simulink model "Dijkstra_Optimization_2"  (R2015b)
settings: Solver=FixedStepDiscrete  SolverMode=SingleTasking  StartTime=0.0  StopTime=10e-5  RelTol=1e-3
libraries: shlslibv1 x995
(part 4 of 6)

== system Dijkstra_Optimization_2/Dijkstra/Subsystem12/Subsystem15/Min_index ==
  dout_sub : Inport
  doutsp_sub : Inport  Port=2
  Comparator1 : shlslibv1/Math Functions/Comparator  syn_comp_opr=a==b  syn_comp_const=on  syn_comp_val=0  syn_en_se=off  synBlockType=primitive  synLatency=0  synBlockId=14
  Comparator2 : shlslibv1/Math Functions/Comparator  syn_comp_opr=a<=b  syn_comp_const=off  syn_comp_val=0  syn_en_se=off  synBlockType=primitive  synLatency=0  synBlockId=14
  Constant4 : shlslibv1/Sources/Constant  syn_cst_val=64  syn_cst_format=Automatic  syn_cst_wl=1  syn_cst_fl=0  syn_cst_dt=unsigned  syn_cst_rnd=on  syn_cst_st=-1  synBlockType=primitive  synLatency=0  synBlockId=15
  Convert1 : shlslibv1/Signal Operations/Convert  syn_preshift_opr=none  syn_preshift_bits=0  syn_preshift_val=0  syn_out_f=Specify  syn_out_wl=64  syn_out_fl=0  syn_out_dt_sync=unsigned  syn_out_sat=off  syn_out_rnd=Floor (Truncate)  syn_inh_port=off  syn_inh_st=off  syn_inh_stf=1  syn_en_pipe=off  syn_pipe_stg=syn_max_pipeline  syn_flow_ctrl=off  syn_sat_op=off  synBlockType=primitive  synLatency=0  synBlockId=4
  Convert2 : shlslibv1/Signal Operations/Convert  syn_preshift_opr=none  syn_preshift_bits=0  syn_preshift_val=0  syn_out_f=Specify  syn_out_wl=4  syn_out_fl=0  syn_out_dt_sync=unsigned  syn_out_sat=off  syn_out_rnd=Floor (Truncate)  syn_inh_port=off  syn_inh_st=off  syn_inh_stf=1  syn_en_pipe=off  syn_pipe_stg=syn_max_pipeline  syn_flow_ctrl=off  syn_sat_op=off  synBlockType=primitive  synLatency=0  synBlockId=4
  Mux : shlslibv1/Signal Operations/Mux  syn_in_nb=2  syn_out_f=Full Precision  syn_out_wl=11  syn_out_fl=52  syn_out_dt=unsigned  syn_en_se=off  synBlockType=primitive  synLatency=0  synBlockId=16
  Switch7 : shlslibv1/Signal Operations/Switch  switchCriteria=u2 != Threshold  switchThresh=0  synBlockType=custom  synLatency=0
  dist10 : shlslibv1/Sources/Sequence  syn_seq_vec=[1 0 0 0 ]  syn_seq_wl=4  syn_seq_fl=0  syn_seq_dt=unsigned  syn_rst_port=off  syn_en_port=off  syn_seq_st=1/(4e6)  synBlockType=custom  synLatency=1
  dist9 : shlslibv1/Sources/Sequence  syn_seq_vec=[0 1 2 3]  syn_seq_wl=4  syn_seq_fl=0  syn_seq_dt=unsigned  syn_rst_port=off  syn_en_port=off  syn_seq_st=1/(4e6)  synBlockType=custom  synLatency=1
  min : shlslibv1/Signal Operations/Mux  syn_in_nb=2  syn_out_f=Full Precision  syn_out_wl=11  syn_out_fl=52  syn_out_dt=unsigned  syn_en_se=off  synBlockType=primitive  synLatency=0  synBlockId=16
  min3 : shlslibv1/Memories/Delay  syn_delay_val=2  synBlockType=primitive  synLatency=2  synBlockId=104
  min4 : shlslibv1/Memories/Delay  syn_delay_val=1  synBlockType=primitive  synLatency=1  synBlockId=104
  min5 : shlslibv1/Memories/Delay  syn_delay_val=1  synBlockType=primitive  synLatency=1  synBlockId=104
  min6 : shlslibv1/Memories/Delay  syn_delay_val=2  synBlockType=primitive  synLatency=2  synBlockId=104
  min_index : shlslibv1/Signal Operations/Mux  syn_in_nb=2  syn_out_f=Full Precision  syn_out_wl=11  syn_out_fl=52  syn_out_dt=unsigned  syn_en_se=off  synBlockType=primitive  synLatency=0  synBlockId=16
  min_sub : Outport
  min_index_sub : Outport  Port=2
  wires:
  min3/1 -> min_index/3
  Comparator1/1 -> Mux/3
  Mux/1 -> Convert2/1
  min/1 -> Convert1/1, min_sub/1
  min_index/1 -> min_index_sub/1, min5/1
  dist9/1 -> min3/1
  dist10/1 -> min6/1
  dout_sub/1 -> Comparator2/1, min/3
  doutsp_sub/1 -> Comparator1/1
  min5/1 -> min_index/2
  Constant4/1 -> Switch7/1
  min6/1 -> Switch7/2
  Switch7/1 -> min/2, Comparator2/2
  min4/1 -> Switch7/3
  Convert2/1 -> min/1, min_index/1
  Convert1/1 -> min4/1
  Comparator2/1 -> Mux/2, Mux/1

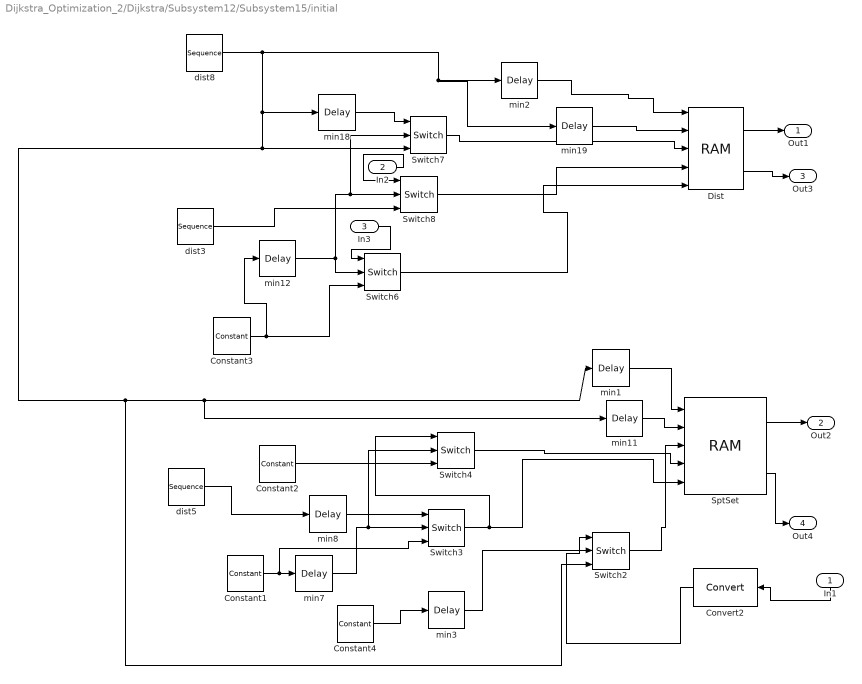
== system Dijkstra_Optimization_2/Dijkstra/Subsystem12/Subsystem15/initial ==
  In1 : Inport
  In2 : Inport  Port=2
  In3 : Inport  Port=3
  Constant1 : shlslibv1/Sources/Constant  syn_cst_val=1  syn_cst_format=Automatic  syn_cst_wl=1  syn_cst_fl=0  syn_cst_dt=unsigned  syn_cst_rnd=on  syn_cst_st=-1  synBlockType=primitive  synLatency=0  synBlockId=15
  Constant2 : shlslibv1/Sources/Constant  syn_cst_val=0  syn_cst_format=Automatic  syn_cst_wl=1  syn_cst_fl=0  syn_cst_dt=unsigned  syn_cst_rnd=on  syn_cst_st=-1  synBlockType=primitive  synLatency=0  synBlockId=15
  Constant3 : shlslibv1/Sources/Constant  syn_cst_val=1  syn_cst_format=Automatic  syn_cst_wl=1  syn_cst_fl=0  syn_cst_dt=unsigned  syn_cst_rnd=on  syn_cst_st=-1  synBlockType=primitive  synLatency=0  synBlockId=15
  Constant4 : shlslibv1/Sources/Constant  syn_cst_val=1  syn_cst_format=Automatic  syn_cst_wl=1  syn_cst_fl=0  syn_cst_dt=unsigned  syn_cst_rnd=on  syn_cst_st=-1  synBlockType=primitive  synLatency=0  synBlockId=15
  Convert2 : shlslibv1/Signal Operations/Convert  syn_preshift_opr=none  syn_preshift_bits=0  syn_preshift_val=0  syn_out_f=Specify  syn_out_wl=4  syn_out_fl=0  syn_out_dt_sync=unsigned  syn_out_sat=off  syn_out_rnd=Floor (Truncate)  syn_inh_port=off  syn_inh_st=off  syn_inh_stf=1  syn_en_pipe=off  syn_pipe_stg=syn_max_pipeline  syn_flow_ctrl=off  syn_sat_op=off  synBlockType=primitive  synLatency=0  synBlockId=4
  "Dist " : shlslibv1/Memories/RAM  syn_ram_depth=4  syn_read_nb=2  syn_write_nb=1  syn_rw_nb=0  syn_corereset=off  syn_localreset=off  syn_initial_val=0  syn_enable_port=off  syn_rrst_port=off  syn_renable_port=off  syn_wac=Write priorization  syn_rac=Cross-port write-first  syn_init_val=0  synBlockType=primitive  synLatency=1  synBlockId=111  syn_spec_init=on
  SptSet : shlslibv1/Memories/RAM  syn_ram_depth=4  syn_read_nb=2  syn_write_nb=1  syn_rw_nb=0  syn_corereset=off  syn_localreset=off  syn_initial_val=0  syn_enable_port=off  syn_rrst_port=off  syn_renable_port=off  syn_wac=Write priorization  syn_rac=Cross-port write-first  syn_init_val=0  synBlockType=primitive  synLatency=1  synBlockId=111  syn_spec_init=on
  Switch{2..4,6..8} (6 alike) : shlslibv1/Signal Operations/Switch  switchCriteria=u2 != Threshold  switchThresh=0  synBlockType=custom  synLatency=0
  dist3 : shlslibv1/Sources/Sequence  syn_seq_vec=[0 64 64 64]  syn_seq_wl=100  syn_seq_fl=0  syn_seq_dt=unsigned  syn_rst_port=off  syn_en_port=off  syn_seq_st=1/(4e6)  synBlockType=custom  synLatency=1
  dist5 : shlslibv1/Sources/Sequence  syn_seq_vec=[0 0 0 1 0 0 0 0 ]  syn_seq_wl=4  syn_seq_fl=0  syn_seq_dt=unsigned  syn_rst_port=off  syn_en_port=off  syn_seq_st=1/(4e6)  synBlockType=custom  synLatency=1
  dist8 : shlslibv1/Sources/Sequence  syn_seq_vec=[0 1 2 3]  syn_seq_wl=4  syn_seq_fl=0  syn_seq_dt=unsigned  syn_rst_port=off  syn_en_port=off  syn_seq_st=1/(4e6)  synBlockType=custom  synLatency=1
  min1 : shlslibv1/Memories/Delay  syn_delay_val=1  synBlockType=primitive  synLatency=1  synBlockId=104
  min{3,7,11..12,19} (5 alike) : shlslibv1/Memories/Delay  syn_delay_val=5  synBlockType=primitive  synLatency=5  synBlockId=104
  min18 : shlslibv1/Memories/Delay  syn_delay_val=6  synBlockType=primitive  synLatency=6  synBlockId=104
  min2 : shlslibv1/Memories/Delay  syn_delay_val=1  synBlockType=primitive  synLatency=1  synBlockId=104
  min8 : shlslibv1/Memories/Delay  syn_delay_val=2  synBlockType=primitive  synLatency=2  synBlockId=104
  Out1 : Outport
  Out2 : Outport  Port=2
  Out3 : Outport  Port=3
  Out4 : Outport  Port=4
  wires:
  In1/1 -> Convert2/1
  In3/1 -> Switch6/1
  In2/1 -> Switch8/1
  min1/1 -> SptSet/1
  min2/1 -> "Dist "/1
  "Dist "/1 -> Out1/1
  SptSet/1 -> Out2/1
  min3/1 -> Switch2/2
  Switch4/1 -> SptSet/4
  Convert2/1 -> Switch2/1
  dist8/1 -> Switch7/3, Switch2/3, min11/1, min1/1, min18/1, min19/1, min2/1
  Constant1/1 -> Switch3/3, min7/1
  Switch3/1 -> Switch4/1, SptSet/5
  Constant2/1 -> Switch4/3
  min7/1 -> Switch4/2, Switch3/2
  dist5/1 -> min8/1
  min8/1 -> Switch3/1
  Switch2/1 -> SptSet/3
  min11/1 -> SptSet/2
  min12/1 -> Switch6/2, Switch8/2, Switch7/2
  Constant3/1 -> Switch6/3, min12/1
  Switch6/1 -> "Dist "/5
  dist3/1 -> Switch8/3
  Switch8/1 -> "Dist "/4
  min18/1 -> Switch7/1
  Switch7/1 -> "Dist "/3
  min19/1 -> "Dist "/2
  Constant4/1 -> min3/1
  SptSet/2 -> Out4/1
  "Dist "/2 -> Out3/1

== system Dijkstra_Optimization_2/Dijkstra/Subsystem12/Subsystem15/min_distance ==
  In1 : Inport
  In2 : Inport  Port=2
  In3 : Inport  Port=3
  In4 : Inport  Port=4
  In5 : Inport  Port=5
  In6 : Inport  Port=6
  In7 : Inport  Port=7
  In8 : Inport  Port=8
  Add1 : shlslibv1/Math Functions/Add  syn_add_opr=++  syn_out_f=Full Precision  syn_out_wl=16  syn_out_fl=8  syn_out_dt=signed  syn_out_sat=off  syn_out_rnd=Floor (Truncate)  synBlockType=primitive  synLatency=0  synBlockId=96  syn_sum_of_rows=off  syn_inh_port=off  syn_inh_st=on  syn_inh_stf=1  syn_en_pipe=off  syn_pipe_stg=syn_max_pipeline  syn_flow_ctrl=off
  Binary Logic1 : shlslibv1/Math Functions/Binary Logic  syn_binlog_exp=a&b&c&d  synBlockType=primitive  synLatency=0  synBlockId=13
  Convert1 : shlslibv1/Signal Operations/Convert  syn_preshift_opr=none  syn_preshift_bits=0  syn_preshift_val=0  syn_out_f=Specify  syn_out_wl=50  syn_out_fl=0  syn_out_dt_sync=unsigned  syn_out_sat=off  syn_out_rnd=Floor (Truncate)  syn_inh_port=off  syn_inh_st=off  syn_inh_stf=1  syn_en_pipe=off  syn_pipe_stg=syn_max_pipeline  syn_flow_ctrl=off  syn_sat_op=off  synBlockType=primitive  synLatency=0  synBlockId=4
  Convert3 : shlslibv1/Signal Operations/Convert  syn_preshift_opr=none  syn_preshift_bits=0  syn_preshift_val=0  syn_out_f=Specify  syn_out_wl=50  syn_out_fl=0  syn_out_dt_sync=unsigned  syn_out_sat=off  syn_out_rnd=Floor (Truncate)  syn_inh_port=off  syn_inh_st=off  syn_inh_stf=1  syn_en_pipe=off  syn_pipe_stg=syn_max_pipeline  syn_flow_ctrl=off  syn_sat_op=off  synBlockType=primitive  synLatency=0  synBlockId=4
  Mux2 : shlslibv1/Signal Operations/Mux  syn_in_nb=4  syn_out_f=Full Precision  syn_out_wl=11  syn_out_fl=52  syn_out_dt=unsigned  syn_en_se=off  synBlockType=primitive  synLatency=0  synBlockId=16
  "dist[u]  INT_MAX " : shlslibv1/Math Functions/Comparator  syn_comp_opr=a!=b  syn_comp_const=on  syn_comp_val=64  syn_en_se=off  synBlockType=primitive  synLatency=0  synBlockId=14
  dist[u][u][v]  dist[v] : shlslibv1/Math Functions/Comparator  syn_comp_opr=a<b  syn_comp_const=off  syn_comp_val=64  syn_en_se=off  synBlockType=primitive  synLatency=0  synBlockId=14
  graph[u][v] : shlslibv1/Math Functions/Comparator  syn_comp_opr=a!=b  syn_comp_const=on  syn_comp_val=0  syn_en_se=off  synBlockType=primitive  synLatency=0  synBlockId=14
  "v]\t" : shlslibv1/Math Functions/Comparator  syn_comp_opr=a==b  syn_comp_const=on  syn_comp_val=0  syn_en_se=off  synBlockType=primitive  synLatency=0  synBlockId=14
  Out1 : Outport
  Out2 : Outport  Port=2
  wires:
  In5/1 -> Mux2/2
  In6/1 -> Mux2/3
  dist[u][u][v]  dist[v]/1 -> Binary Logic1/1
  "dist[u]  INT_MAX "/1 -> Binary Logic1/2
  graph[u][v]/1 -> Binary Logic1/3
  Add1/1 -> Convert3/1, dist[u][u][v]  dist[v]/1
  Binary Logic1/1 -> Convert1/1
  "v]\t"/1 -> Binary Logic1/4
  Mux2/1 -> Add1/2, graph[u][v]/1
  In4/1 -> "v]\t"/1
  Convert3/1 -> Out1/1
  Convert1/1 -> Out2/1
  In1/1 -> dist[u][u][v]  dist[v]/2
  In2/1 -> "dist[u]  INT_MAX "/1, Add1/1
  In3/1 -> Mux2/1
  In8/1 -> Mux2/5
  In7/1 -> Mux2/4

== system Dijkstra_Optimization_2/Dijkstra/Subsystem13/Subsystem16/Delay ==
  In1 : Inport
  In2 : Inport  Port=2
  Switch10 : shlslibv1/Signal Operations/Switch  switchCriteria=u2 != Threshold  switchThresh=0  synBlockType=custom  synLatency=0
  Switch5 : shlslibv1/Signal Operations/Switch  switchCriteria=u2 != Threshold  switchThresh=0  synBlockType=custom  synLatency=0
  dist6 : shlslibv1/Sources/Sequence  syn_seq_vec=[0 0 0 1 0 0 0 0 ]  syn_seq_wl=4  syn_seq_fl=0  syn_seq_dt=unsigned  syn_rst_port=off  syn_en_port=off  syn_seq_st=1/(4e6)  synBlockType=custom  synLatency=1
  min10 : shlslibv1/Memories/Delay  syn_delay_val=2  synBlockType=primitive  synLatency=2  synBlockId=104
  min4 : shlslibv1/Memories/Delay  syn_delay_val=1  synBlockType=primitive  synLatency=1  synBlockId=104
  min9 : shlslibv1/Memories/Delay  syn_delay_val=1  synBlockType=primitive  synLatency=1  synBlockId=104
  Out1 : Outport
  Out2 : Outport  Port=2
  wires:
  In2/1 -> Switch5/1
  dist6/1 -> min10/1
  min10/1 -> Switch5/2, Switch10/2
  In1/1 -> Switch10/1
  Switch10/1 -> Out1/1, min9/1
  Switch5/1 -> min4/1
  min9/1 -> Switch10/3
  min4/1 -> Switch5/3, Out2/1

== system Dijkstra_Optimization_2/Dijkstra/Subsystem13/Subsystem16/Input ==
  In1 : Inport
  In2 : Inport  Port=2
  In3 : Inport  Port=3
  In4 : Inport  Port=4
  Constant5 : shlslibv1/Sources/Constant  syn_cst_val=1  syn_cst_format=Automatic  syn_cst_wl=1  syn_cst_fl=0  syn_cst_dt=unsigned  syn_cst_rnd=on  syn_cst_st=-1  synBlockType=primitive  synLatency=0  synBlockId=15
  Constant6 : shlslibv1/Sources/Constant  syn_cst_val=0  syn_cst_format=Automatic  syn_cst_wl=1  syn_cst_fl=0  syn_cst_dt=unsigned  syn_cst_rnd=on  syn_cst_st=-1  synBlockType=primitive  synLatency=0  synBlockId=15
  Graph{0..3} (4 alike) : shlslibv1/Memories/RAM  syn_ram_depth=4  syn_read_nb=1  syn_write_nb=1  syn_rw_nb=0  syn_corereset=off  syn_localreset=off  syn_initial_val=0  syn_enable_port=off  syn_rrst_port=off  syn_renable_port=off  syn_wac=Write priorization  syn_rac=Cross-port write-first  syn_init_val=0  synBlockType=primitive  synLatency=1  synBlockId=111  syn_spec_init=on
  Switch1 : shlslibv1/Signal Operations/Switch  switchCriteria=u2 != Threshold  switchThresh=0  synBlockType=custom  synLatency=0
  dist9 : shlslibv1/Sources/Sequence  syn_seq_vec=[0 1 2 3 ]  syn_seq_wl=4  syn_seq_fl=0  syn_seq_dt=unsigned  syn_rst_port=off  syn_en_port=off  syn_seq_st=1/(4e6)  synBlockType=custom  synLatency=1
  min14 : shlslibv1/Memories/Delay  syn_delay_val=5  synBlockType=primitive  synLatency=5  synBlockId=104
  min15 : shlslibv1/Memories/Delay  syn_delay_val=5  synBlockType=primitive  synLatency=5  synBlockId=104
  Out1 : Outport
  Out2 : Outport  Port=2
  Out3 : Outport  Port=3
  Out4 : Outport  Port=4
  wires:
  Constant5/1 -> min14/1, Switch1/3
  min14/1 -> Switch1/2
  Switch1/1 -> Graph3/4, Graph2/4, Graph1/4, Graph0/4
  Constant6/1 -> Switch1/1
  In1/1 -> Graph0/3
  In2/1 -> Graph1/3
  In3/1 -> Graph2/3
  In4/1 -> Graph3/3
  dist9/1 -> min15/1, Graph3/2, Graph2/2, Graph1/2, Graph0/2
  min15/1 -> Graph2/1, Graph3/1, Graph1/1, Graph0/1
  Graph0/1 -> Out1/1
  Graph3/1 -> Out4/1
  Graph2/1 -> Out3/1
  Graph1/1 -> Out2/1

== system Dijkstra_Optimization_2/Dijkstra/Subsystem13/Subsystem16/Min_index ==
  dout_sub : Inport
  doutsp_sub : Inport  Port=2
  Comparator1 : shlslibv1/Math Functions/Comparator  syn_comp_opr=a==b  syn_comp_const=on  syn_comp_val=0  syn_en_se=off  synBlockType=primitive  synLatency=0  synBlockId=14
  Comparator2 : shlslibv1/Math Functions/Comparator  syn_comp_opr=a<=b  syn_comp_const=off  syn_comp_val=0  syn_en_se=off  synBlockType=primitive  synLatency=0  synBlockId=14
  Constant4 : shlslibv1/Sources/Constant  syn_cst_val=64  syn_cst_format=Automatic  syn_cst_wl=1  syn_cst_fl=0  syn_cst_dt=unsigned  syn_cst_rnd=on  syn_cst_st=-1  synBlockType=primitive  synLatency=0  synBlockId=15
  Convert1 : shlslibv1/Signal Operations/Convert  syn_preshift_opr=none  syn_preshift_bits=0  syn_preshift_val=0  syn_out_f=Specify  syn_out_wl=64  syn_out_fl=0  syn_out_dt_sync=unsigned  syn_out_sat=off  syn_out_rnd=Floor (Truncate)  syn_inh_port=off  syn_inh_st=off  syn_inh_stf=1  syn_en_pipe=off  syn_pipe_stg=syn_max_pipeline  syn_flow_ctrl=off  syn_sat_op=off  synBlockType=primitive  synLatency=0  synBlockId=4
  Convert2 : shlslibv1/Signal Operations/Convert  syn_preshift_opr=none  syn_preshift_bits=0  syn_preshift_val=0  syn_out_f=Specify  syn_out_wl=4  syn_out_fl=0  syn_out_dt_sync=unsigned  syn_out_sat=off  syn_out_rnd=Floor (Truncate)  syn_inh_port=off  syn_inh_st=off  syn_inh_stf=1  syn_en_pipe=off  syn_pipe_stg=syn_max_pipeline  syn_flow_ctrl=off  syn_sat_op=off  synBlockType=primitive  synLatency=0  synBlockId=4
  Mux : shlslibv1/Signal Operations/Mux  syn_in_nb=2  syn_out_f=Full Precision  syn_out_wl=11  syn_out_fl=52  syn_out_dt=unsigned  syn_en_se=off  synBlockType=primitive  synLatency=0  synBlockId=16
  Switch7 : shlslibv1/Signal Operations/Switch  switchCriteria=u2 != Threshold  switchThresh=0  synBlockType=custom  synLatency=0
  dist10 : shlslibv1/Sources/Sequence  syn_seq_vec=[1 0 0 0 ]  syn_seq_wl=4  syn_seq_fl=0  syn_seq_dt=unsigned  syn_rst_port=off  syn_en_port=off  syn_seq_st=1/(4e6)  synBlockType=custom  synLatency=1
  dist9 : shlslibv1/Sources/Sequence  syn_seq_vec=[0 1 2 3]  syn_seq_wl=4  syn_seq_fl=0  syn_seq_dt=unsigned  syn_rst_port=off  syn_en_port=off  syn_seq_st=1/(4e6)  synBlockType=custom  synLatency=1
  min : shlslibv1/Signal Operations/Mux  syn_in_nb=2  syn_out_f=Full Precision  syn_out_wl=11  syn_out_fl=52  syn_out_dt=unsigned  syn_en_se=off  synBlockType=primitive  synLatency=0  synBlockId=16
  min3 : shlslibv1/Memories/Delay  syn_delay_val=2  synBlockType=primitive  synLatency=2  synBlockId=104
  min4 : shlslibv1/Memories/Delay  syn_delay_val=1  synBlockType=primitive  synLatency=1  synBlockId=104
  min5 : shlslibv1/Memories/Delay  syn_delay_val=1  synBlockType=primitive  synLatency=1  synBlockId=104
  min6 : shlslibv1/Memories/Delay  syn_delay_val=2  synBlockType=primitive  synLatency=2  synBlockId=104
  min_index : shlslibv1/Signal Operations/Mux  syn_in_nb=2  syn_out_f=Full Precision  syn_out_wl=11  syn_out_fl=52  syn_out_dt=unsigned  syn_en_se=off  synBlockType=primitive  synLatency=0  synBlockId=16
  min_sub : Outport
  min_index_sub : Outport  Port=2
  wires:
  min3/1 -> min_index/3
  Comparator1/1 -> Mux/3
  Mux/1 -> Convert2/1
  min/1 -> Convert1/1, min_sub/1
  min_index/1 -> min_index_sub/1, min5/1
  dist9/1 -> min3/1
  dist10/1 -> min6/1
  dout_sub/1 -> Comparator2/1, min/3
  doutsp_sub/1 -> Comparator1/1
  min5/1 -> min_index/2
  Constant4/1 -> Switch7/1
  min6/1 -> Switch7/2
  Switch7/1 -> min/2, Comparator2/2
  min4/1 -> Switch7/3
  Convert2/1 -> min/1, min_index/1
  Convert1/1 -> min4/1
  Comparator2/1 -> Mux/2, Mux/1

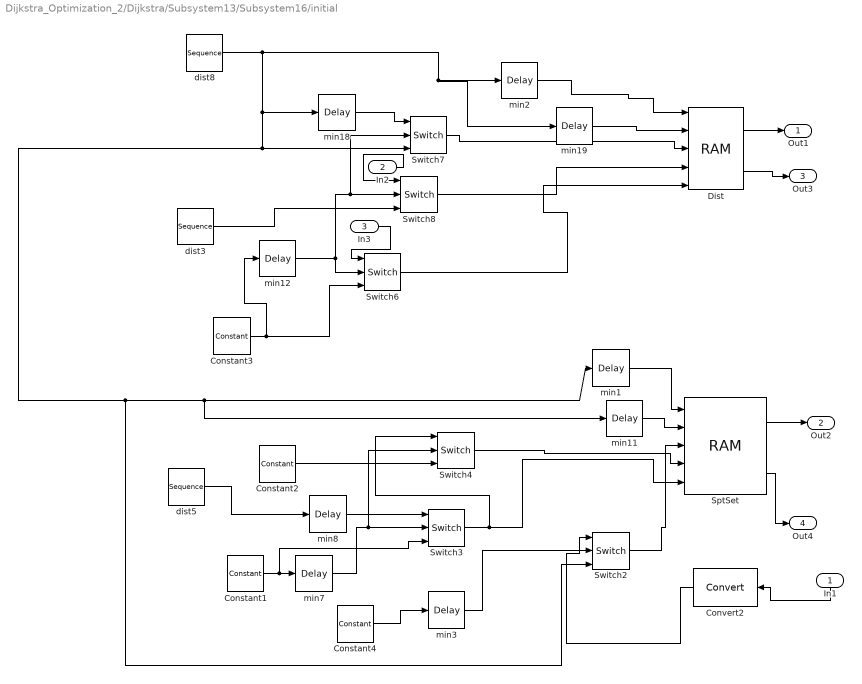
== system Dijkstra_Optimization_2/Dijkstra/Subsystem13/Subsystem16/initial ==
  In1 : Inport
  In2 : Inport  Port=2
  In3 : Inport  Port=3
  Constant1 : shlslibv1/Sources/Constant  syn_cst_val=1  syn_cst_format=Automatic  syn_cst_wl=1  syn_cst_fl=0  syn_cst_dt=unsigned  syn_cst_rnd=on  syn_cst_st=-1  synBlockType=primitive  synLatency=0  synBlockId=15
  Constant2 : shlslibv1/Sources/Constant  syn_cst_val=0  syn_cst_format=Automatic  syn_cst_wl=1  syn_cst_fl=0  syn_cst_dt=unsigned  syn_cst_rnd=on  syn_cst_st=-1  synBlockType=primitive  synLatency=0  synBlockId=15
  Constant3 : shlslibv1/Sources/Constant  syn_cst_val=1  syn_cst_format=Automatic  syn_cst_wl=1  syn_cst_fl=0  syn_cst_dt=unsigned  syn_cst_rnd=on  syn_cst_st=-1  synBlockType=primitive  synLatency=0  synBlockId=15
  Constant4 : shlslibv1/Sources/Constant  syn_cst_val=1  syn_cst_format=Automatic  syn_cst_wl=1  syn_cst_fl=0  syn_cst_dt=unsigned  syn_cst_rnd=on  syn_cst_st=-1  synBlockType=primitive  synLatency=0  synBlockId=15
  Convert2 : shlslibv1/Signal Operations/Convert  syn_preshift_opr=none  syn_preshift_bits=0  syn_preshift_val=0  syn_out_f=Specify  syn_out_wl=4  syn_out_fl=0  syn_out_dt_sync=unsigned  syn_out_sat=off  syn_out_rnd=Floor (Truncate)  syn_inh_port=off  syn_inh_st=off  syn_inh_stf=1  syn_en_pipe=off  syn_pipe_stg=syn_max_pipeline  syn_flow_ctrl=off  syn_sat_op=off  synBlockType=primitive  synLatency=0  synBlockId=4
  "Dist " : shlslibv1/Memories/RAM  syn_ram_depth=4  syn_read_nb=2  syn_write_nb=1  syn_rw_nb=0  syn_corereset=off  syn_localreset=off  syn_initial_val=0  syn_enable_port=off  syn_rrst_port=off  syn_renable_port=off  syn_wac=Write priorization  syn_rac=Cross-port write-first  syn_init_val=0  synBlockType=primitive  synLatency=1  synBlockId=111  syn_spec_init=on
  SptSet : shlslibv1/Memories/RAM  syn_ram_depth=4  syn_read_nb=2  syn_write_nb=1  syn_rw_nb=0  syn_corereset=off  syn_localreset=off  syn_initial_val=0  syn_enable_port=off  syn_rrst_port=off  syn_renable_port=off  syn_wac=Write priorization  syn_rac=Cross-port write-first  syn_init_val=0  synBlockType=primitive  synLatency=1  synBlockId=111  syn_spec_init=on
  Switch{2..4,6..8} (6 alike) : shlslibv1/Signal Operations/Switch  switchCriteria=u2 != Threshold  switchThresh=0  synBlockType=custom  synLatency=0
  dist3 : shlslibv1/Sources/Sequence  syn_seq_vec=[0 64 64 64]  syn_seq_wl=100  syn_seq_fl=0  syn_seq_dt=unsigned  syn_rst_port=off  syn_en_port=off  syn_seq_st=1/(4e6)  synBlockType=custom  synLatency=1
  dist5 : shlslibv1/Sources/Sequence  syn_seq_vec=[0 0 0 1 0 0 0 0 ]  syn_seq_wl=4  syn_seq_fl=0  syn_seq_dt=unsigned  syn_rst_port=off  syn_en_port=off  syn_seq_st=1/(4e6)  synBlockType=custom  synLatency=1
  dist8 : shlslibv1/Sources/Sequence  syn_seq_vec=[0 1 2 3]  syn_seq_wl=4  syn_seq_fl=0  syn_seq_dt=unsigned  syn_rst_port=off  syn_en_port=off  syn_seq_st=1/(4e6)  synBlockType=custom  synLatency=1
  min1 : shlslibv1/Memories/Delay  syn_delay_val=1  synBlockType=primitive  synLatency=1  synBlockId=104
  min{3,7,11..12,19} (5 alike) : shlslibv1/Memories/Delay  syn_delay_val=5  synBlockType=primitive  synLatency=5  synBlockId=104
  min18 : shlslibv1/Memories/Delay  syn_delay_val=6  synBlockType=primitive  synLatency=6  synBlockId=104
  min2 : shlslibv1/Memories/Delay  syn_delay_val=1  synBlockType=primitive  synLatency=1  synBlockId=104
  min8 : shlslibv1/Memories/Delay  syn_delay_val=2  synBlockType=primitive  synLatency=2  synBlockId=104
  Out1 : Outport
  Out2 : Outport  Port=2
  Out3 : Outport  Port=3
  Out4 : Outport  Port=4
  wires:
  In1/1 -> Convert2/1
  In3/1 -> Switch6/1
  In2/1 -> Switch8/1
  min1/1 -> SptSet/1
  min2/1 -> "Dist "/1
  "Dist "/1 -> Out1/1
  SptSet/1 -> Out2/1
  min3/1 -> Switch2/2
  Switch4/1 -> SptSet/4
  Convert2/1 -> Switch2/1
  dist8/1 -> Switch7/3, Switch2/3, min11/1, min1/1, min18/1, min19/1, min2/1
  Constant1/1 -> Switch3/3, min7/1
  Switch3/1 -> Switch4/1, SptSet/5
  Constant2/1 -> Switch4/3
  min7/1 -> Switch4/2, Switch3/2
  dist5/1 -> min8/1
  min8/1 -> Switch3/1
  Switch2/1 -> SptSet/3
  min11/1 -> SptSet/2
  min12/1 -> Switch6/2, Switch8/2, Switch7/2
  Constant3/1 -> Switch6/3, min12/1
  Switch6/1 -> "Dist "/5
  dist3/1 -> Switch8/3
  Switch8/1 -> "Dist "/4
  min18/1 -> Switch7/1
  Switch7/1 -> "Dist "/3
  min19/1 -> "Dist "/2
  Constant4/1 -> min3/1
  SptSet/2 -> Out4/1
  "Dist "/2 -> Out3/1

== system Dijkstra_Optimization_2/Dijkstra/Subsystem13/Subsystem16/min_distance ==
  In1 : Inport
  In2 : Inport  Port=2
  In3 : Inport  Port=3
  In4 : Inport  Port=4
  In5 : Inport  Port=5
  In6 : Inport  Port=6
  In7 : Inport  Port=7
  In8 : Inport  Port=8
  Add1 : shlslibv1/Math Functions/Add  syn_add_opr=++  syn_out_f=Full Precision  syn_out_wl=16  syn_out_fl=8  syn_out_dt=signed  syn_out_sat=off  syn_out_rnd=Floor (Truncate)  synBlockType=primitive  synLatency=0  synBlockId=96  syn_sum_of_rows=off  syn_inh_port=off  syn_inh_st=on  syn_inh_stf=1  syn_en_pipe=off  syn_pipe_stg=syn_max_pipeline  syn_flow_ctrl=off
  Binary Logic1 : shlslibv1/Math Functions/Binary Logic  syn_binlog_exp=a&b&c&d  synBlockType=primitive  synLatency=0  synBlockId=13
  Convert1 : shlslibv1/Signal Operations/Convert  syn_preshift_opr=none  syn_preshift_bits=0  syn_preshift_val=0  syn_out_f=Specify  syn_out_wl=50  syn_out_fl=0  syn_out_dt_sync=unsigned  syn_out_sat=off  syn_out_rnd=Floor (Truncate)  syn_inh_port=off  syn_inh_st=off  syn_inh_stf=1  syn_en_pipe=off  syn_pipe_stg=syn_max_pipeline  syn_flow_ctrl=off  syn_sat_op=off  synBlockType=primitive  synLatency=0  synBlockId=4
  Convert3 : shlslibv1/Signal Operations/Convert  syn_preshift_opr=none  syn_preshift_bits=0  syn_preshift_val=0  syn_out_f=Specify  syn_out_wl=50  syn_out_fl=0  syn_out_dt_sync=unsigned  syn_out_sat=off  syn_out_rnd=Floor (Truncate)  syn_inh_port=off  syn_inh_st=off  syn_inh_stf=1  syn_en_pipe=off  syn_pipe_stg=syn_max_pipeline  syn_flow_ctrl=off  syn_sat_op=off  synBlockType=primitive  synLatency=0  synBlockId=4
  Mux2 : shlslibv1/Signal Operations/Mux  syn_in_nb=4  syn_out_f=Full Precision  syn_out_wl=11  syn_out_fl=52  syn_out_dt=unsigned  syn_en_se=off  synBlockType=primitive  synLatency=0  synBlockId=16
  "dist[u]  INT_MAX " : shlslibv1/Math Functions/Comparator  syn_comp_opr=a!=b  syn_comp_const=on  syn_comp_val=64  syn_en_se=off  synBlockType=primitive  synLatency=0  synBlockId=14
  dist[u][u][v]  dist[v] : shlslibv1/Math Functions/Comparator  syn_comp_opr=a<b  syn_comp_const=off  syn_comp_val=64  syn_en_se=off  synBlockType=primitive  synLatency=0  synBlockId=14
  graph[u][v] : shlslibv1/Math Functions/Comparator  syn_comp_opr=a!=b  syn_comp_const=on  syn_comp_val=0  syn_en_se=off  synBlockType=primitive  synLatency=0  synBlockId=14
  "v]\t" : shlslibv1/Math Functions/Comparator  syn_comp_opr=a==b  syn_comp_const=on  syn_comp_val=0  syn_en_se=off  synBlockType=primitive  synLatency=0  synBlockId=14
  Out1 : Outport
  Out2 : Outport  Port=2
  wires:
  In5/1 -> Mux2/2
  In6/1 -> Mux2/3
  dist[u][u][v]  dist[v]/1 -> Binary Logic1/1
  "dist[u]  INT_MAX "/1 -> Binary Logic1/2
  graph[u][v]/1 -> Binary Logic1/3
  Add1/1 -> Convert3/1, dist[u][u][v]  dist[v]/1
  Binary Logic1/1 -> Convert1/1
  "v]\t"/1 -> Binary Logic1/4
  Mux2/1 -> Add1/2, graph[u][v]/1
  In4/1 -> "v]\t"/1
  Convert3/1 -> Out1/1
  Convert1/1 -> Out2/1
  In1/1 -> dist[u][u][v]  dist[v]/2
  In2/1 -> "dist[u]  INT_MAX "/1, Add1/1
  In3/1 -> Mux2/1
  In8/1 -> Mux2/5
  In7/1 -> Mux2/4

== system Dijkstra_Optimization_2/Dijkstra/Subsystem14/Subsystem28/Delay ==
  In1 : Inport
  In2 : Inport  Port=2
  Switch10 : shlslibv1/Signal Operations/Switch  switchCriteria=u2 != Threshold  switchThresh=0  synBlockType=custom  synLatency=0
  Switch5 : shlslibv1/Signal Operations/Switch  switchCriteria=u2 != Threshold  switchThresh=0  synBlockType=custom  synLatency=0
  dist6 : shlslibv1/Sources/Sequence  syn_seq_vec=[0 0 0 1 0 0 0 0 ]  syn_seq_wl=4  syn_seq_fl=0  syn_seq_dt=unsigned  syn_rst_port=off  syn_en_port=off  syn_seq_st=1/(4e6)  synBlockType=custom  synLatency=1
  min10 : shlslibv1/Memories/Delay  syn_delay_val=2  synBlockType=primitive  synLatency=2  synBlockId=104
  min4 : shlslibv1/Memories/Delay  syn_delay_val=1  synBlockType=primitive  synLatency=1  synBlockId=104
  min9 : shlslibv1/Memories/Delay  syn_delay_val=1  synBlockType=primitive  synLatency=1  synBlockId=104
  Out1 : Outport
  Out2 : Outport  Port=2
  wires:
  In2/1 -> Switch5/1
  dist6/1 -> min10/1
  min10/1 -> Switch5/2, Switch10/2
  In1/1 -> Switch10/1
  Switch10/1 -> Out1/1, min9/1
  Switch5/1 -> min4/1
  min9/1 -> Switch10/3
  min4/1 -> Switch5/3, Out2/1

== system Dijkstra_Optimization_2/Dijkstra/Subsystem14/Subsystem28/Input ==
  In1 : Inport
  In2 : Inport  Port=2
  In3 : Inport  Port=3
  In4 : Inport  Port=4
  Constant5 : shlslibv1/Sources/Constant  syn_cst_val=1  syn_cst_format=Automatic  syn_cst_wl=1  syn_cst_fl=0  syn_cst_dt=unsigned  syn_cst_rnd=on  syn_cst_st=-1  synBlockType=primitive  synLatency=0  synBlockId=15
  Constant6 : shlslibv1/Sources/Constant  syn_cst_val=0  syn_cst_format=Automatic  syn_cst_wl=1  syn_cst_fl=0  syn_cst_dt=unsigned  syn_cst_rnd=on  syn_cst_st=-1  synBlockType=primitive  synLatency=0  synBlockId=15
  Graph{0..3} (4 alike) : shlslibv1/Memories/RAM  syn_ram_depth=4  syn_read_nb=1  syn_write_nb=1  syn_rw_nb=0  syn_corereset=off  syn_localreset=off  syn_initial_val=0  syn_enable_port=off  syn_rrst_port=off  syn_renable_port=off  syn_wac=Write priorization  syn_rac=Cross-port write-first  syn_init_val=0  synBlockType=primitive  synLatency=1  synBlockId=111  syn_spec_init=on
  Switch1 : shlslibv1/Signal Operations/Switch  switchCriteria=u2 != Threshold  switchThresh=0  synBlockType=custom  synLatency=0
  dist9 : shlslibv1/Sources/Sequence  syn_seq_vec=[0 1 2 3 ]  syn_seq_wl=4  syn_seq_fl=0  syn_seq_dt=unsigned  syn_rst_port=off  syn_en_port=off  syn_seq_st=1/(4e6)  synBlockType=custom  synLatency=1
  min14 : shlslibv1/Memories/Delay  syn_delay_val=5  synBlockType=primitive  synLatency=5  synBlockId=104
  min15 : shlslibv1/Memories/Delay  syn_delay_val=5  synBlockType=primitive  synLatency=5  synBlockId=104
  Out1 : Outport
  Out2 : Outport  Port=2
  Out3 : Outport  Port=3
  Out4 : Outport  Port=4
  wires:
  Constant5/1 -> min14/1, Switch1/3
  min14/1 -> Switch1/2
  Switch1/1 -> Graph3/4, Graph2/4, Graph1/4, Graph0/4
  Constant6/1 -> Switch1/1
  In1/1 -> Graph0/3
  In2/1 -> Graph1/3
  In3/1 -> Graph2/3
  In4/1 -> Graph3/3
  dist9/1 -> min15/1, Graph3/2, Graph2/2, Graph1/2, Graph0/2
  min15/1 -> Graph2/1, Graph3/1, Graph1/1, Graph0/1
  Graph0/1 -> Out1/1
  Graph3/1 -> Out4/1
  Graph2/1 -> Out3/1
  Graph1/1 -> Out2/1

== system Dijkstra_Optimization_2/Dijkstra/Subsystem14/Subsystem28/Min_index ==
  dout_sub : Inport
  doutsp_sub : Inport  Port=2
  Comparator1 : shlslibv1/Math Functions/Comparator  syn_comp_opr=a==b  syn_comp_const=on  syn_comp_val=0  syn_en_se=off  synBlockType=primitive  synLatency=0  synBlockId=14
  Comparator2 : shlslibv1/Math Functions/Comparator  syn_comp_opr=a<=b  syn_comp_const=off  syn_comp_val=0  syn_en_se=off  synBlockType=primitive  synLatency=0  synBlockId=14
  Constant4 : shlslibv1/Sources/Constant  syn_cst_val=64  syn_cst_format=Automatic  syn_cst_wl=1  syn_cst_fl=0  syn_cst_dt=unsigned  syn_cst_rnd=on  syn_cst_st=-1  synBlockType=primitive  synLatency=0  synBlockId=15
  Convert1 : shlslibv1/Signal Operations/Convert  syn_preshift_opr=none  syn_preshift_bits=0  syn_preshift_val=0  syn_out_f=Specify  syn_out_wl=64  syn_out_fl=0  syn_out_dt_sync=unsigned  syn_out_sat=off  syn_out_rnd=Floor (Truncate)  syn_inh_port=off  syn_inh_st=off  syn_inh_stf=1  syn_en_pipe=off  syn_pipe_stg=syn_max_pipeline  syn_flow_ctrl=off  syn_sat_op=off  synBlockType=primitive  synLatency=0  synBlockId=4
  Convert2 : shlslibv1/Signal Operations/Convert  syn_preshift_opr=none  syn_preshift_bits=0  syn_preshift_val=0  syn_out_f=Specify  syn_out_wl=4  syn_out_fl=0  syn_out_dt_sync=unsigned  syn_out_sat=off  syn_out_rnd=Floor (Truncate)  syn_inh_port=off  syn_inh_st=off  syn_inh_stf=1  syn_en_pipe=off  syn_pipe_stg=syn_max_pipeline  syn_flow_ctrl=off  syn_sat_op=off  synBlockType=primitive  synLatency=0  synBlockId=4
  Mux : shlslibv1/Signal Operations/Mux  syn_in_nb=2  syn_out_f=Full Precision  syn_out_wl=11  syn_out_fl=52  syn_out_dt=unsigned  syn_en_se=off  synBlockType=primitive  synLatency=0  synBlockId=16
  Switch7 : shlslibv1/Signal Operations/Switch  switchCriteria=u2 != Threshold  switchThresh=0  synBlockType=custom  synLatency=0
  dist10 : shlslibv1/Sources/Sequence  syn_seq_vec=[1 0 0 0 ]  syn_seq_wl=4  syn_seq_fl=0  syn_seq_dt=unsigned  syn_rst_port=off  syn_en_port=off  syn_seq_st=1/(4e6)  synBlockType=custom  synLatency=1
  dist9 : shlslibv1/Sources/Sequence  syn_seq_vec=[0 1 2 3]  syn_seq_wl=4  syn_seq_fl=0  syn_seq_dt=unsigned  syn_rst_port=off  syn_en_port=off  syn_seq_st=1/(4e6)  synBlockType=custom  synLatency=1
  min : shlslibv1/Signal Operations/Mux  syn_in_nb=2  syn_out_f=Full Precision  syn_out_wl=11  syn_out_fl=52  syn_out_dt=unsigned  syn_en_se=off  synBlockType=primitive  synLatency=0  synBlockId=16
  min3 : shlslibv1/Memories/Delay  syn_delay_val=2  synBlockType=primitive  synLatency=2  synBlockId=104
  min4 : shlslibv1/Memories/Delay  syn_delay_val=1  synBlockType=primitive  synLatency=1  synBlockId=104
  min5 : shlslibv1/Memories/Delay  syn_delay_val=1  synBlockType=primitive  synLatency=1  synBlockId=104
  min6 : shlslibv1/Memories/Delay  syn_delay_val=2  synBlockType=primitive  synLatency=2  synBlockId=104
  min_index : shlslibv1/Signal Operations/Mux  syn_in_nb=2  syn_out_f=Full Precision  syn_out_wl=11  syn_out_fl=52  syn_out_dt=unsigned  syn_en_se=off  synBlockType=primitive  synLatency=0  synBlockId=16
  min_sub : Outport
  min_index_sub : Outport  Port=2
  wires:
  min3/1 -> min_index/3
  Comparator1/1 -> Mux/3
  Mux/1 -> Convert2/1
  min/1 -> Convert1/1, min_sub/1
  min_index/1 -> min_index_sub/1, min5/1
  dist9/1 -> min3/1
  dist10/1 -> min6/1
  dout_sub/1 -> Comparator2/1, min/3
  doutsp_sub/1 -> Comparator1/1
  min5/1 -> min_index/2
  Constant4/1 -> Switch7/1
  min6/1 -> Switch7/2
  Switch7/1 -> min/2, Comparator2/2
  min4/1 -> Switch7/3
  Convert2/1 -> min/1, min_index/1
  Convert1/1 -> min4/1
  Comparator2/1 -> Mux/2, Mux/1

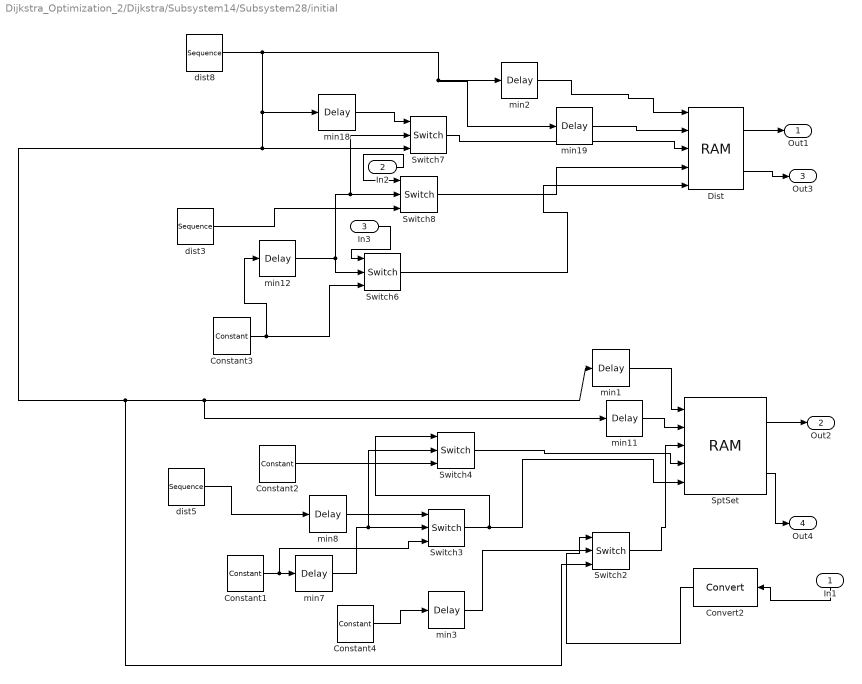
== system Dijkstra_Optimization_2/Dijkstra/Subsystem14/Subsystem28/initial ==
  In1 : Inport
  In2 : Inport  Port=2
  In3 : Inport  Port=3
  Constant1 : shlslibv1/Sources/Constant  syn_cst_val=1  syn_cst_format=Automatic  syn_cst_wl=1  syn_cst_fl=0  syn_cst_dt=unsigned  syn_cst_rnd=on  syn_cst_st=-1  synBlockType=primitive  synLatency=0  synBlockId=15
  Constant2 : shlslibv1/Sources/Constant  syn_cst_val=0  syn_cst_format=Automatic  syn_cst_wl=1  syn_cst_fl=0  syn_cst_dt=unsigned  syn_cst_rnd=on  syn_cst_st=-1  synBlockType=primitive  synLatency=0  synBlockId=15
  Constant3 : shlslibv1/Sources/Constant  syn_cst_val=1  syn_cst_format=Automatic  syn_cst_wl=1  syn_cst_fl=0  syn_cst_dt=unsigned  syn_cst_rnd=on  syn_cst_st=-1  synBlockType=primitive  synLatency=0  synBlockId=15
  Constant4 : shlslibv1/Sources/Constant  syn_cst_val=1  syn_cst_format=Automatic  syn_cst_wl=1  syn_cst_fl=0  syn_cst_dt=unsigned  syn_cst_rnd=on  syn_cst_st=-1  synBlockType=primitive  synLatency=0  synBlockId=15
  Convert2 : shlslibv1/Signal Operations/Convert  syn_preshift_opr=none  syn_preshift_bits=0  syn_preshift_val=0  syn_out_f=Specify  syn_out_wl=4  syn_out_fl=0  syn_out_dt_sync=unsigned  syn_out_sat=off  syn_out_rnd=Floor (Truncate)  syn_inh_port=off  syn_inh_st=off  syn_inh_stf=1  syn_en_pipe=off  syn_pipe_stg=syn_max_pipeline  syn_flow_ctrl=off  syn_sat_op=off  synBlockType=primitive  synLatency=0  synBlockId=4
  "Dist " : shlslibv1/Memories/RAM  syn_ram_depth=4  syn_read_nb=2  syn_write_nb=1  syn_rw_nb=0  syn_corereset=off  syn_localreset=off  syn_initial_val=0  syn_enable_port=off  syn_rrst_port=off  syn_renable_port=off  syn_wac=Write priorization  syn_rac=Cross-port write-first  syn_init_val=0  synBlockType=primitive  synLatency=1  synBlockId=111  syn_spec_init=on
  SptSet : shlslibv1/Memories/RAM  syn_ram_depth=4  syn_read_nb=2  syn_write_nb=1  syn_rw_nb=0  syn_corereset=off  syn_localreset=off  syn_initial_val=0  syn_enable_port=off  syn_rrst_port=off  syn_renable_port=off  syn_wac=Write priorization  syn_rac=Cross-port write-first  syn_init_val=0  synBlockType=primitive  synLatency=1  synBlockId=111  syn_spec_init=on
  Switch{2..4,6..8} (6 alike) : shlslibv1/Signal Operations/Switch  switchCriteria=u2 != Threshold  switchThresh=0  synBlockType=custom  synLatency=0
  dist3 : shlslibv1/Sources/Sequence  syn_seq_vec=[0 64 64 64]  syn_seq_wl=100  syn_seq_fl=0  syn_seq_dt=unsigned  syn_rst_port=off  syn_en_port=off  syn_seq_st=1/(4e6)  synBlockType=custom  synLatency=1
  dist5 : shlslibv1/Sources/Sequence  syn_seq_vec=[0 0 0 1 0 0 0 0 ]  syn_seq_wl=4  syn_seq_fl=0  syn_seq_dt=unsigned  syn_rst_port=off  syn_en_port=off  syn_seq_st=1/(4e6)  synBlockType=custom  synLatency=1
  dist8 : shlslibv1/Sources/Sequence  syn_seq_vec=[0 1 2 3]  syn_seq_wl=4  syn_seq_fl=0  syn_seq_dt=unsigned  syn_rst_port=off  syn_en_port=off  syn_seq_st=1/(4e6)  synBlockType=custom  synLatency=1
  min1 : shlslibv1/Memories/Delay  syn_delay_val=1  synBlockType=primitive  synLatency=1  synBlockId=104
  min{3,7,11..12,19} (5 alike) : shlslibv1/Memories/Delay  syn_delay_val=5  synBlockType=primitive  synLatency=5  synBlockId=104
  min18 : shlslibv1/Memories/Delay  syn_delay_val=6  synBlockType=primitive  synLatency=6  synBlockId=104
  min2 : shlslibv1/Memories/Delay  syn_delay_val=1  synBlockType=primitive  synLatency=1  synBlockId=104
  min8 : shlslibv1/Memories/Delay  syn_delay_val=2  synBlockType=primitive  synLatency=2  synBlockId=104
  Out1 : Outport
  Out2 : Outport  Port=2
  Out3 : Outport  Port=3
  Out4 : Outport  Port=4
  wires:
  In1/1 -> Convert2/1
  In3/1 -> Switch6/1
  In2/1 -> Switch8/1
  min1/1 -> SptSet/1
  min2/1 -> "Dist "/1
  "Dist "/1 -> Out1/1
  SptSet/1 -> Out2/1
  min3/1 -> Switch2/2
  Switch4/1 -> SptSet/4
  Convert2/1 -> Switch2/1
  dist8/1 -> Switch7/3, Switch2/3, min11/1, min1/1, min18/1, min19/1, min2/1
  Constant1/1 -> Switch3/3, min7/1
  Switch3/1 -> Switch4/1, SptSet/5
  Constant2/1 -> Switch4/3
  min7/1 -> Switch4/2, Switch3/2
  dist5/1 -> min8/1
  min8/1 -> Switch3/1
  Switch2/1 -> SptSet/3
  min11/1 -> SptSet/2
  min12/1 -> Switch6/2, Switch8/2, Switch7/2
  Constant3/1 -> Switch6/3, min12/1
  Switch6/1 -> "Dist "/5
  dist3/1 -> Switch8/3
  Switch8/1 -> "Dist "/4
  min18/1 -> Switch7/1
  Switch7/1 -> "Dist "/3
  min19/1 -> "Dist "/2
  Constant4/1 -> min3/1
  SptSet/2 -> Out4/1
  "Dist "/2 -> Out3/1

== system Dijkstra_Optimization_2/Dijkstra/Subsystem14/Subsystem28/min_distance ==
  In1 : Inport
  In2 : Inport  Port=2
  In3 : Inport  Port=3
  In4 : Inport  Port=4
  In5 : Inport  Port=5
  In6 : Inport  Port=6
  In7 : Inport  Port=7
  In8 : Inport  Port=8
  Add1 : shlslibv1/Math Functions/Add  syn_add_opr=++  syn_out_f=Full Precision  syn_out_wl=16  syn_out_fl=8  syn_out_dt=signed  syn_out_sat=off  syn_out_rnd=Floor (Truncate)  synBlockType=primitive  synLatency=0  synBlockId=96  syn_sum_of_rows=off  syn_inh_port=off  syn_inh_st=on  syn_inh_stf=1  syn_en_pipe=off  syn_pipe_stg=syn_max_pipeline  syn_flow_ctrl=off
  Binary Logic1 : shlslibv1/Math Functions/Binary Logic  syn_binlog_exp=a&b&c&d  synBlockType=primitive  synLatency=0  synBlockId=13
  Convert1 : shlslibv1/Signal Operations/Convert  syn_preshift_opr=none  syn_preshift_bits=0  syn_preshift_val=0  syn_out_f=Specify  syn_out_wl=50  syn_out_fl=0  syn_out_dt_sync=unsigned  syn_out_sat=off  syn_out_rnd=Floor (Truncate)  syn_inh_port=off  syn_inh_st=off  syn_inh_stf=1  syn_en_pipe=off  syn_pipe_stg=syn_max_pipeline  syn_flow_ctrl=off  syn_sat_op=off  synBlockType=primitive  synLatency=0  synBlockId=4
  Convert3 : shlslibv1/Signal Operations/Convert  syn_preshift_opr=none  syn_preshift_bits=0  syn_preshift_val=0  syn_out_f=Specify  syn_out_wl=50  syn_out_fl=0  syn_out_dt_sync=unsigned  syn_out_sat=off  syn_out_rnd=Floor (Truncate)  syn_inh_port=off  syn_inh_st=off  syn_inh_stf=1  syn_en_pipe=off  syn_pipe_stg=syn_max_pipeline  syn_flow_ctrl=off  syn_sat_op=off  synBlockType=primitive  synLatency=0  synBlockId=4
  Mux2 : shlslibv1/Signal Operations/Mux  syn_in_nb=4  syn_out_f=Full Precision  syn_out_wl=11  syn_out_fl=52  syn_out_dt=unsigned  syn_en_se=off  synBlockType=primitive  synLatency=0  synBlockId=16
  "dist[u]  INT_MAX " : shlslibv1/Math Functions/Comparator  syn_comp_opr=a!=b  syn_comp_const=on  syn_comp_val=64  syn_en_se=off  synBlockType=primitive  synLatency=0  synBlockId=14
  dist[u][u][v]  dist[v] : shlslibv1/Math Functions/Comparator  syn_comp_opr=a<b  syn_comp_const=off  syn_comp_val=64  syn_en_se=off  synBlockType=primitive  synLatency=0  synBlockId=14
  graph[u][v] : shlslibv1/Math Functions/Comparator  syn_comp_opr=a!=b  syn_comp_const=on  syn_comp_val=0  syn_en_se=off  synBlockType=primitive  synLatency=0  synBlockId=14
  "v]\t" : shlslibv1/Math Functions/Comparator  syn_comp_opr=a==b  syn_comp_const=on  syn_comp_val=0  syn_en_se=off  synBlockType=primitive  synLatency=0  synBlockId=14
  Out1 : Outport
  Out2 : Outport  Port=2
  wires:
  In5/1 -> Mux2/2
  In6/1 -> Mux2/3
  dist[u][u][v]  dist[v]/1 -> Binary Logic1/1
  "dist[u]  INT_MAX "/1 -> Binary Logic1/2
  graph[u][v]/1 -> Binary Logic1/3
  Add1/1 -> Convert3/1, dist[u][u][v]  dist[v]/1
  Binary Logic1/1 -> Convert1/1
  "v]\t"/1 -> Binary Logic1/4
  Mux2/1 -> Add1/2, graph[u][v]/1
  In4/1 -> "v]\t"/1
  Convert3/1 -> Out1/1
  Convert1/1 -> Out2/1
  In1/1 -> dist[u][u][v]  dist[v]/2
  In2/1 -> "dist[u]  INT_MAX "/1, Add1/1
  In3/1 -> Mux2/1
  In8/1 -> Mux2/5
  In7/1 -> Mux2/4

== system Dijkstra_Optimization_2/Dijkstra/Subsystem15/Subsystem22/Delay ==
  In1 : Inport
  In2 : Inport  Port=2
  Switch10 : shlslibv1/Signal Operations/Switch  switchCriteria=u2 != Threshold  switchThresh=0  synBlockType=custom  synLatency=0
  Switch5 : shlslibv1/Signal Operations/Switch  switchCriteria=u2 != Threshold  switchThresh=0  synBlockType=custom  synLatency=0
  dist6 : shlslibv1/Sources/Sequence  syn_seq_vec=[0 0 0 1 0 0 0 0 ]  syn_seq_wl=4  syn_seq_fl=0  syn_seq_dt=unsigned  syn_rst_port=off  syn_en_port=off  syn_seq_st=1/(4e6)  synBlockType=custom  synLatency=1
  min10 : shlslibv1/Memories/Delay  syn_delay_val=2  synBlockType=primitive  synLatency=2  synBlockId=104
  min4 : shlslibv1/Memories/Delay  syn_delay_val=1  synBlockType=primitive  synLatency=1  synBlockId=104
  min9 : shlslibv1/Memories/Delay  syn_delay_val=1  synBlockType=primitive  synLatency=1  synBlockId=104
  Out1 : Outport
  Out2 : Outport  Port=2
  wires:
  In2/1 -> Switch5/1
  dist6/1 -> min10/1
  min10/1 -> Switch5/2, Switch10/2
  In1/1 -> Switch10/1
  Switch10/1 -> Out1/1, min9/1
  Switch5/1 -> min4/1
  min9/1 -> Switch10/3
  min4/1 -> Switch5/3, Out2/1

== system Dijkstra_Optimization_2/Dijkstra/Subsystem15/Subsystem22/Input ==
  In1 : Inport
  In2 : Inport  Port=2
  In3 : Inport  Port=3
  In4 : Inport  Port=4
  Constant5 : shlslibv1/Sources/Constant  syn_cst_val=1  syn_cst_format=Automatic  syn_cst_wl=1  syn_cst_fl=0  syn_cst_dt=unsigned  syn_cst_rnd=on  syn_cst_st=-1  synBlockType=primitive  synLatency=0  synBlockId=15
  Constant6 : shlslibv1/Sources/Constant  syn_cst_val=0  syn_cst_format=Automatic  syn_cst_wl=1  syn_cst_fl=0  syn_cst_dt=unsigned  syn_cst_rnd=on  syn_cst_st=-1  synBlockType=primitive  synLatency=0  synBlockId=15
  Graph{0..3} (4 alike) : shlslibv1/Memories/RAM  syn_ram_depth=4  syn_read_nb=1  syn_write_nb=1  syn_rw_nb=0  syn_corereset=off  syn_localreset=off  syn_initial_val=0  syn_enable_port=off  syn_rrst_port=off  syn_renable_port=off  syn_wac=Write priorization  syn_rac=Cross-port write-first  syn_init_val=0  synBlockType=primitive  synLatency=1  synBlockId=111  syn_spec_init=on
  Switch1 : shlslibv1/Signal Operations/Switch  switchCriteria=u2 != Threshold  switchThresh=0  synBlockType=custom  synLatency=0
  dist9 : shlslibv1/Sources/Sequence  syn_seq_vec=[0 1 2 3 ]  syn_seq_wl=4  syn_seq_fl=0  syn_seq_dt=unsigned  syn_rst_port=off  syn_en_port=off  syn_seq_st=1/(4e6)  synBlockType=custom  synLatency=1
  min14 : shlslibv1/Memories/Delay  syn_delay_val=5  synBlockType=primitive  synLatency=5  synBlockId=104
  min15 : shlslibv1/Memories/Delay  syn_delay_val=5  synBlockType=primitive  synLatency=5  synBlockId=104
  Out1 : Outport
  Out2 : Outport  Port=2
  Out3 : Outport  Port=3
  Out4 : Outport  Port=4
  wires:
  Constant5/1 -> min14/1, Switch1/3
  min14/1 -> Switch1/2
  Switch1/1 -> Graph3/4, Graph2/4, Graph1/4, Graph0/4
  Constant6/1 -> Switch1/1
  In1/1 -> Graph0/3
  In2/1 -> Graph1/3
  In3/1 -> Graph2/3
  In4/1 -> Graph3/3
  dist9/1 -> min15/1, Graph3/2, Graph2/2, Graph1/2, Graph0/2
  min15/1 -> Graph2/1, Graph3/1, Graph1/1, Graph0/1
  Graph0/1 -> Out1/1
  Graph3/1 -> Out4/1
  Graph2/1 -> Out3/1
  Graph1/1 -> Out2/1

== system Dijkstra_Optimization_2/Dijkstra/Subsystem15/Subsystem22/Min_index ==
  dout_sub : Inport
  doutsp_sub : Inport  Port=2
  Comparator1 : shlslibv1/Math Functions/Comparator  syn_comp_opr=a==b  syn_comp_const=on  syn_comp_val=0  syn_en_se=off  synBlockType=primitive  synLatency=0  synBlockId=14
  Comparator2 : shlslibv1/Math Functions/Comparator  syn_comp_opr=a<=b  syn_comp_const=off  syn_comp_val=0  syn_en_se=off  synBlockType=primitive  synLatency=0  synBlockId=14
  Constant4 : shlslibv1/Sources/Constant  syn_cst_val=64  syn_cst_format=Automatic  syn_cst_wl=1  syn_cst_fl=0  syn_cst_dt=unsigned  syn_cst_rnd=on  syn_cst_st=-1  synBlockType=primitive  synLatency=0  synBlockId=15
  Convert1 : shlslibv1/Signal Operations/Convert  syn_preshift_opr=none  syn_preshift_bits=0  syn_preshift_val=0  syn_out_f=Specify  syn_out_wl=64  syn_out_fl=0  syn_out_dt_sync=unsigned  syn_out_sat=off  syn_out_rnd=Floor (Truncate)  syn_inh_port=off  syn_inh_st=off  syn_inh_stf=1  syn_en_pipe=off  syn_pipe_stg=syn_max_pipeline  syn_flow_ctrl=off  syn_sat_op=off  synBlockType=primitive  synLatency=0  synBlockId=4
  Convert2 : shlslibv1/Signal Operations/Convert  syn_preshift_opr=none  syn_preshift_bits=0  syn_preshift_val=0  syn_out_f=Specify  syn_out_wl=4  syn_out_fl=0  syn_out_dt_sync=unsigned  syn_out_sat=off  syn_out_rnd=Floor (Truncate)  syn_inh_port=off  syn_inh_st=off  syn_inh_stf=1  syn_en_pipe=off  syn_pipe_stg=syn_max_pipeline  syn_flow_ctrl=off  syn_sat_op=off  synBlockType=primitive  synLatency=0  synBlockId=4
  Mux : shlslibv1/Signal Operations/Mux  syn_in_nb=2  syn_out_f=Full Precision  syn_out_wl=11  syn_out_fl=52  syn_out_dt=unsigned  syn_en_se=off  synBlockType=primitive  synLatency=0  synBlockId=16
  Switch7 : shlslibv1/Signal Operations/Switch  switchCriteria=u2 != Threshold  switchThresh=0  synBlockType=custom  synLatency=0
  dist10 : shlslibv1/Sources/Sequence  syn_seq_vec=[1 0 0 0 ]  syn_seq_wl=4  syn_seq_fl=0  syn_seq_dt=unsigned  syn_rst_port=off  syn_en_port=off  syn_seq_st=1/(4e6)  synBlockType=custom  synLatency=1
  dist9 : shlslibv1/Sources/Sequence  syn_seq_vec=[0 1 2 3]  syn_seq_wl=4  syn_seq_fl=0  syn_seq_dt=unsigned  syn_rst_port=off  syn_en_port=off  syn_seq_st=1/(4e6)  synBlockType=custom  synLatency=1
  min : shlslibv1/Signal Operations/Mux  syn_in_nb=2  syn_out_f=Full Precision  syn_out_wl=11  syn_out_fl=52  syn_out_dt=unsigned  syn_en_se=off  synBlockType=primitive  synLatency=0  synBlockId=16
  min3 : shlslibv1/Memories/Delay  syn_delay_val=2  synBlockType=primitive  synLatency=2  synBlockId=104
  min4 : shlslibv1/Memories/Delay  syn_delay_val=1  synBlockType=primitive  synLatency=1  synBlockId=104
  min5 : shlslibv1/Memories/Delay  syn_delay_val=1  synBlockType=primitive  synLatency=1  synBlockId=104
  min6 : shlslibv1/Memories/Delay  syn_delay_val=2  synBlockType=primitive  synLatency=2  synBlockId=104
  min_index : shlslibv1/Signal Operations/Mux  syn_in_nb=2  syn_out_f=Full Precision  syn_out_wl=11  syn_out_fl=52  syn_out_dt=unsigned  syn_en_se=off  synBlockType=primitive  synLatency=0  synBlockId=16
  min_sub : Outport
  min_index_sub : Outport  Port=2
  wires:
  min3/1 -> min_index/3
  Comparator1/1 -> Mux/3
  Mux/1 -> Convert2/1
  min/1 -> Convert1/1, min_sub/1
  min_index/1 -> min_index_sub/1, min5/1
  dist9/1 -> min3/1
  dist10/1 -> min6/1
  dout_sub/1 -> Comparator2/1, min/3
  doutsp_sub/1 -> Comparator1/1
  min5/1 -> min_index/2
  Constant4/1 -> Switch7/1
  min6/1 -> Switch7/2
  Switch7/1 -> min/2, Comparator2/2
  min4/1 -> Switch7/3
  Convert2/1 -> min/1, min_index/1
  Convert1/1 -> min4/1
  Comparator2/1 -> Mux/2, Mux/1
